simulink model "main_sim_generalized"  (R2024a)
settings: Solver=VariableStepAuto  StartTime=0.0  StopTime=Tsim  FixedStep=simStepSize  RelTol=1e-3
undefined symbols (not defined in the file): A_amp, B_para, f_d, f_hz, ForceDist, L_t, mmp_fir_coeff, mmp_iir_coeff, p_off, Ps_sys, Pz_sys, Qcvx_FIR, Qcvx_IIR, Qcvx_sim, SensorNoise, T_cs, T_fs, T_ss, Ts, Tu, w_k, w_k_IIR
libraries: cstblocks x6
settings Model: Creator=tomli  LastModifiedBy=tomli
settings RTWCC: GPUComputeCapability=3.5

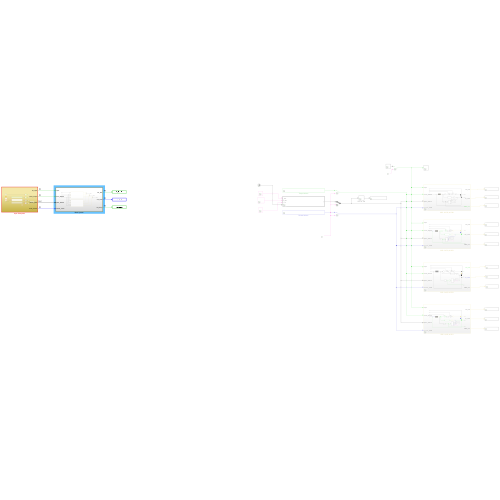
[thumbnail: Simulink's stored preview of the top-level diagram]
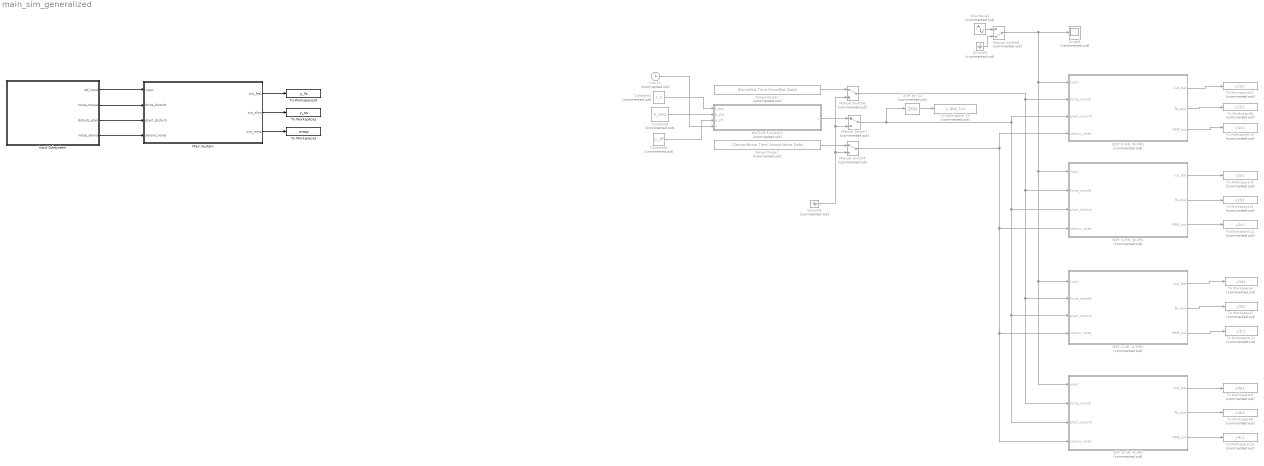
== system main_sim_generalized ==
  Clock1 : Clock  Commented=on
  Constant1 : Constant  Commented=on  Value=f_d
  Constant2 : Constant  Commented=on  Value=A_amp
  Constant3 : Constant  Commented=on  Value=p_off
  Ground3 : Ground  Commented=on
  Ground4 : Ground  Commented=on
  Input Subsystem : Subsystem
  MATLAB Function1 : MATLAB Function  Commented=on  TreatAsAtomicUnit=on
  Main System : Subsystem
  Manual Switch4 : ManualSwitch  Commented=on
  Manual Switch6 : ManualSwitch  Commented=on
  Manual Switch7 : ManualSwitch  Commented=on
  Manual Switch8 : ManualSwitch  Commented=on  CurrentSetting=0
  "SDP: Q-FIR, W-FIR1" : Subsystem  Commented=on
  "SDP: Q-FIR, W-IIR1" : Subsystem  Commented=on
  "SDP: Q-IIR, W-FIR1" : Subsystem  Commented=on
  "SDP: Q-IIR, W-IIR1" : Subsystem  Commented=on
  Scope1 : Scope  Commented=on
  Sensor Noise1 : FromWorkspace  Commented=on  VariableName=[SensorNoise.Time,SensorNoise.Data]  SampleTime=SensorNoise.Ts  Interpolate=off  ZeroCross=off  OutputAfterFinalValue=Setting to zero
  Sine Wave1 : Sin  Commented=on  SampleTime=Ts
  To Workspace 10 : ToWorkspace  Commented=on  VariableName=y1c1  SaveFormat=Structure With Time  SampleTime=Tu
      settings: MaxDataPoints=Inf
  To Workspace 11 : ToWorkspace  Commented=on  VariableName=y3c1  SaveFormat=Structure With Time  SampleTime=Tu
      settings: MaxDataPoints=Inf
  To Workspace 12 : ToWorkspace  Commented=on  VariableName=y2c1  SaveFormat=Structure With Time  SampleTime=Tu
      settings: MaxDataPoints=Inf
  To Workspace 13 : ToWorkspace  Commented=on  VariableName=y_dist_Tu1  SaveFormat=Structure With Time  SampleTime=Tu
      settings: MaxDataPoints=Inf
  To Workspace 14 : ToWorkspace  Commented=on  VariableName=y4c1  SaveFormat=Structure With Time  SampleTime=Tu
      settings: MaxDataPoints=Inf
  To Workspace 8 : ToWorkspace  Commented=on  VariableName=y2a1  SaveFormat=Structure With Time  SampleTime=Tu
      settings: MaxDataPoints=Inf
  To Workspace 9 : ToWorkspace  Commented=on  VariableName=y4a1  SaveFormat=Structure With Time  SampleTime=Tu
      settings: MaxDataPoints=Inf
  To Workspace1 : ToWorkspace  VariableName=y_ss  SaveFormat=Structure With Time  SampleTime=-1
  To Workspace10 : ToWorkspace  VariableName=y_fs  SaveFormat=Structure With Time  SampleTime=-1
  To Workspace11 : ToWorkspace  Commented=on  VariableName=y2b1  SaveFormat=Structure With Time  SampleTime=Ts
  To Workspace12 : ToWorkspace  Commented=on  VariableName=y1a1  SaveFormat=Structure With Time  SampleTime=-1
  To Workspace2 : ToWorkspace  VariableName=mmp  SaveFormat=Structure With Time  SampleTime=-1
  To Workspace4 : ToWorkspace  Commented=on  VariableName=y3a1  SaveFormat=Structure With Time  SampleTime=-1
  To Workspace6 : ToWorkspace  Commented=on  VariableName=y1b1  SaveFormat=Structure With Time  SampleTime=-1
  To Workspace7 : ToWorkspace  Commented=on  VariableName=y3b1  SaveFormat=Structure With Time  SampleTime=-1
  To Workspace8 : ToWorkspace  Commented=on  VariableName=y4b1  SaveFormat=Structure With Time  SampleTime=Ts
  Torque Noise1 : FromWorkspace  Commented=on  VariableName=[ForceDist.Time,ForceDist.Data]  SampleTime=ForceDist.Ts  Interpolate=off  ZeroCross=off  OutputAfterFinalValue=Setting to zero
  ZOH at Tu2 : ZeroOrderHold  Commented=on  SampleTime=Tu
  wires:
  Sensor Noise1/1 -> Manual Switch4/1
  "SDP: Q-IIR, W-FIR1"/2(fb_slow) -> To Workspace7/1
  Manual Switch7/1 -> ZOH at Tu2/1, "SDP: Q-IIR, W-IIR1"/3(plant_disturb), "SDP: Q-IIR, W-FIR1"/3(plant_disturb), "SDP: Q-FIR, W-IIR1"/3(plant_disturb), "SDP: Q-FIR, W-FIR1"/3(plant_disturb)
  Manual Switch4/1 -> "SDP: Q-FIR, W-FIR1"/4(sensor_noise), "SDP: Q-IIR, W-IIR1"/4(sensor_noise), "SDP: Q-IIR, W-FIR1"/4(sensor_noise), "SDP: Q-FIR, W-IIR1"/4(sensor_noise)
  "SDP: Q-IIR, W-IIR1"/2(fb_slow) -> To Workspace8/1
  "SDP: Q-FIR, W-FIR1"/2(fb_slow) -> To Workspace6/1
  "SDP: Q-FIR, W-FIR1"/3(MMP_out) -> To Workspace 10/1
  Torque Noise1/1 -> Manual Switch6/1
  Sine Wave1/1 -> Manual Switch8/1
  MATLAB Function1/1(y) -> Manual Switch7/1
  Manual Switch8/1 -> "SDP: Q-IIR, W-IIR1"/1(input), "SDP: Q-IIR, W-FIR1"/1(input), "SDP: Q-FIR, W-IIR1"/1(input), "SDP: Q-FIR, W-FIR1"/1(input), Scope1/1
  "SDP: Q-IIR, W-FIR1"/1(out_fast) -> To Workspace4/1
  "SDP: Q-IIR, W-IIR1"/3(MMP_out) -> To Workspace 14/1
  "SDP: Q-FIR, W-FIR1"/1(out_fast) -> To Workspace12/1
  "SDP: Q-IIR, W-IIR1"/1(out_fast) -> To Workspace 9/1
  Ground4/1 -> Manual Switch8/2
  ZOH at Tu2/1 -> To Workspace 13/1
  "SDP: Q-FIR, W-IIR1"/1(out_fast) -> To Workspace 8/1
  Constant1/1 -> MATLAB Function1/1(f_dist)
  Constant2/1 -> MATLAB Function1/2(A_dist)
  Ground3/1 -> Manual Switch6/2, Manual Switch7/2, Manual Switch4/2
  Clock1/1 -> MATLAB Function1/4(u)
  "SDP: Q-FIR, W-IIR1"/3(MMP_out) -> To Workspace 12/1
  Manual Switch6/1 -> "SDP: Q-IIR, W-IIR1"/2(force_disturb), "SDP: Q-IIR, W-FIR1"/2(force_disturb), "SDP: Q-FIR, W-IIR1"/2(force_disturb), "SDP: Q-FIR, W-FIR1"/2(force_disturb)
  Constant3/1 -> MATLAB Function1/3(p_off)
  "SDP: Q-IIR, W-FIR1"/3(MMP_out) -> To Workspace 11/1
  "SDP: Q-FIR, W-IIR1"/2(fb_slow) -> To Workspace11/1
  Input Subsystem/1(ref_input) -> Main System/1(input)
  Input Subsystem/2(noise_torque) -> Main System/2(force_disturb)
  Input Subsystem/3(disturb_plant) -> Main System/3(plant_disturb)
  Input Subsystem/4(noise_sensor) -> Main System/4(sensor_noise)
  Main System/3(out_mmp) -> To Workspace2/1
  Main System/2(out_slow) -> To Workspace1/1
  Main System/1(out_fast) -> To Workspace10/1

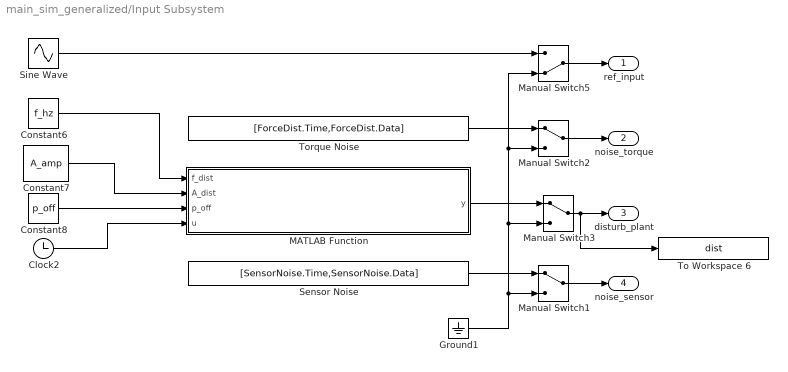
== system main_sim_generalized/Input Subsystem ==
  Clock2 : Clock
  Constant6 : Constant  Value=f_hz
  Constant7 : Constant  Value=A_amp
  Constant8 : Constant  Value=p_off
  Ground1 : Ground
  MATLAB Function : MATLAB Function  TreatAsAtomicUnit=on
  Manual Switch1 : ManualSwitch
  Manual Switch2 : ManualSwitch
  Manual Switch3 : ManualSwitch
  Manual Switch5 : ManualSwitch  CurrentSetting=0
  Sensor Noise : FromWorkspace  VariableName=[SensorNoise.Time,SensorNoise.Data]  SampleTime=SensorNoise.Ts  Interpolate=off  ZeroCross=off  OutputAfterFinalValue=Setting to zero
  Sine Wave : Sin  SampleTime=T_fs
  To Workspace 6 : ToWorkspace  VariableName=dist  SaveFormat=Structure With Time  SampleTime=T_fs
      settings: MaxDataPoints=Inf
  Torque Noise : FromWorkspace  VariableName=[ForceDist.Time,ForceDist.Data]  SampleTime=ForceDist.Ts  Interpolate=off  ZeroCross=off  OutputAfterFinalValue=Setting to zero
  ref_input : Outport
  noise_torque : Outport  Port=2
  disturb_plant : Outport  Port=3
  noise_sensor : Outport  Port=4
  wires:
  Manual Switch1/1 -> noise_sensor/1
  Constant7/1 -> MATLAB Function/2(A_dist)
  Constant8/1 -> MATLAB Function/3(p_off)
  Torque Noise/1 -> Manual Switch2/1
  Ground1/1 -> Manual Switch5/2, Manual Switch2/2, Manual Switch3/2, Manual Switch1/2
  Manual Switch3/1 -> To Workspace 6/1, disturb_plant/1
  Constant6/1 -> MATLAB Function/1(f_dist)
  Sine Wave/1 -> Manual Switch5/1
  MATLAB Function/1(y) -> Manual Switch3/1
  Clock2/1 -> MATLAB Function/4(u)
  Sensor Noise/1 -> Manual Switch1/1
  Manual Switch2/1 -> noise_torque/1
  Manual Switch5/1 -> ref_input/1

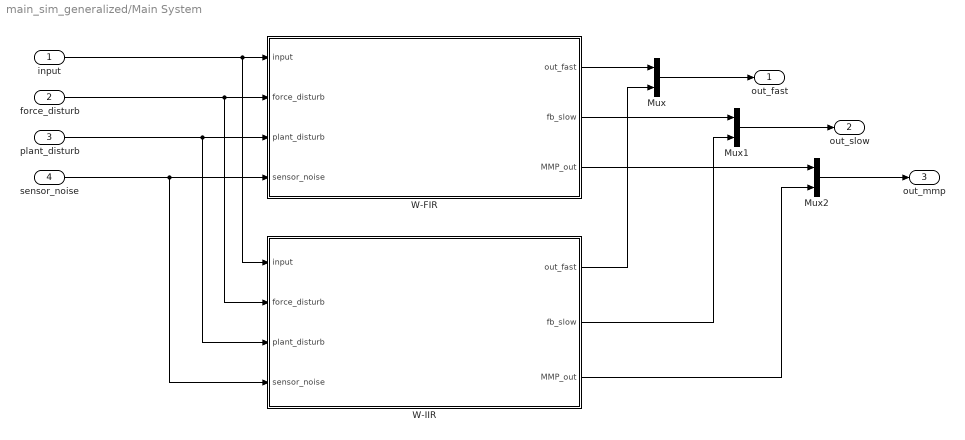
== system main_sim_generalized/Main System ==
  input : Inport
  force_disturb : Inport  Port=2
  plant_disturb : Inport  Port=3
  sensor_noise : Inport  Port=4
  Mux : Mux  Inputs=2
  Mux1 : Mux  Inputs=2
  Mux2 : Mux  Inputs=2
  W-FIR : Subsystem
  W-IIR : Subsystem
  out_fast : Outport
  out_slow : Outport  Port=2
  out_mmp : Outport  Port=3
  wires:
  W-FIR/2(fb_slow) -> Mux1/1
  plant_disturb/1 -> W-IIR/3(plant_disturb), W-FIR/3(plant_disturb)
  W-IIR/2(fb_slow) -> Mux1/2
  Mux1/1 -> out_slow/1
  W-IIR/1(out_fast) -> Mux/2
  sensor_noise/1 -> W-IIR/4(sensor_noise), W-FIR/4(sensor_noise)
  W-FIR/1(out_fast) -> Mux/1
  Mux/1 -> out_fast/1
  Mux2/1 -> out_mmp/1
  force_disturb/1 -> W-IIR/2(force_disturb), W-FIR/2(force_disturb)
  W-FIR/3(MMP_out) -> Mux2/1
  input/1 -> W-IIR/1(input), W-FIR/1(input)
  W-IIR/3(MMP_out) -> Mux2/2

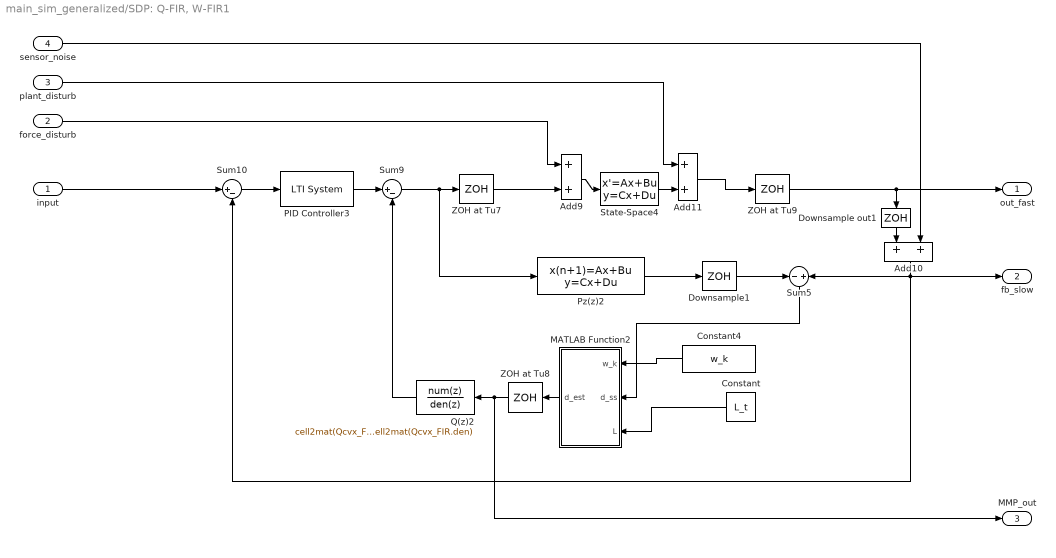
== system main_sim_generalized/SDP: Q-FIR, W-FIR1 ==
  input : Inport
  force_disturb : Inport  Port=2
  plant_disturb : Inport  Port=3
  sensor_noise : Inport  Port=4
  Add10 : Sum
  Add11 : Sum
  Add9 : Sum
  Constant : Constant  Value=L_t
  Constant4 : Constant  Value=w_k
  Downsample out1 : ZeroOrderHold  SampleTime=Ts
  Downsample1 : ZeroOrderHold  SampleTime=Ts
  MATLAB Function2 : MATLAB Function  TreatAsAtomicUnit=on  SystemSampleTime=T_cs
  PID Controller3 : cstblocks/LTI System  sys=Cz  IC=[]  PadeOrder=0
  Pz(z)2 : DiscreteStateSpace  A=Pz_sys.A  B=Pz_sys.B  C=Pz_sys.C  D=Pz_sys.D  SampleTime=Tu
  Q(z)2 : DiscreteTransferFcn  Numerator=cell2mat(Qcvx_FIR.num)  Denominator=cell2mat(Qcvx_FIR.den)  SampleTime=Tu
  State-Space4 : StateSpace  A=Ps_sys.A  B=Ps_sys.B  C=Ps_sys.C  D=Ps_sys.D  InitialCondition=0
  Sum10 : Sum  Inputs=|+-
  Sum5 : Sum  Inputs=-|+
  Sum9 : Sum  Inputs=|+-
  ZOH at Tu7 : ZeroOrderHold  SampleTime=Tu
  ZOH at Tu8 : ZeroOrderHold  SampleTime=Tu
  ZOH at Tu9 : ZeroOrderHold  SampleTime=Tu
  out_fast : Outport
  fb_slow : Outport  Port=2
  MMP_out : Outport  Port=3
  wires:
  ZOH at Tu9/1 -> Downsample out1/1, out_fast/1
  Sum9/1 -> Pz(z)2/1, ZOH at Tu7/1
  State-Space4/1 -> Add11/2
  Constant4/1 -> MATLAB Function2/1(w_k)
  Add10/1 -> Sum5/2, Sum10/2, fb_slow/1
  MATLAB Function2/1(d_est) -> ZOH at Tu8/1
  Add11/1 -> ZOH at Tu9/1
  force_disturb/1 -> Add9/1
  input/1 -> Sum10/1
  Pz(z)2/1 -> Downsample1/1
  ZOH at Tu8/1 -> MMP_out/1, Q(z)2/1
  Sum10/1 -> PID Controller3/1
  Add9/1 -> State-Space4/1
  Q(z)2/1 -> Sum9/2
  ZOH at Tu7/1 -> Add9/2
  Downsample1/1 -> Sum5/1
  Constant/1 -> MATLAB Function2/3(L)
  plant_disturb/1 -> Add11/1
  sensor_noise/1 -> Add10/2
  Downsample out1/1 -> Add10/1
  Sum5/1 -> MATLAB Function2/2(d_ss)
  PID Controller3/1 -> Sum9/1

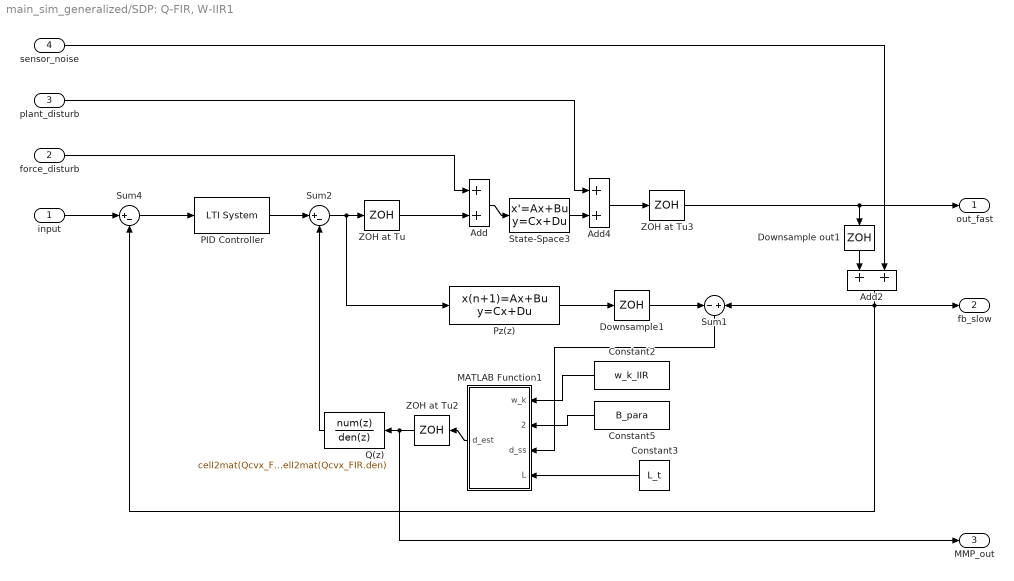
== system main_sim_generalized/SDP: Q-FIR, W-IIR1 ==
  input : Inport
  force_disturb : Inport  Port=2
  plant_disturb : Inport  Port=3
  sensor_noise : Inport  Port=4
  Add : Sum
  Add2 : Sum
  Add4 : Sum
  Constant2 : Constant  Value=w_k_IIR
  Constant3 : Constant  Value=L_t
  Constant5 : Constant  Value=B_para
  Downsample out1 : ZeroOrderHold  SampleTime=Ts
  Downsample1 : ZeroOrderHold  SampleTime=Ts
  MATLAB Function1 : MATLAB Function  TreatAsAtomicUnit=on  SystemSampleTime=T_cs
  PID Controller : cstblocks/LTI System  sys=Cz  IC=[]  PadeOrder=0
  Pz(z) : DiscreteStateSpace  A=Pz_sys.A  B=Pz_sys.B  C=Pz_sys.C  D=Pz_sys.D  SampleTime=Tu
  Q(z) : DiscreteTransferFcn  Numerator=cell2mat(Qcvx_FIR.num)  Denominator=cell2mat(Qcvx_FIR.den)  SampleTime=Tu
  State-Space3 : StateSpace  A=Ps_sys.A  B=Ps_sys.B  C=Ps_sys.C  D=Ps_sys.D  InitialCondition=0
  Sum1 : Sum  Inputs=-|+
  Sum2 : Sum  Inputs=|+-
  Sum4 : Sum  Inputs=|+-
  ZOH at Tu : ZeroOrderHold  SampleTime=Tu
  ZOH at Tu2 : ZeroOrderHold  SampleTime=Tu
  ZOH at Tu3 : ZeroOrderHold  SampleTime=Tu
  out_fast : Outport
  fb_slow : Outport  Port=2
  MMP_out : Outport  Port=3
  wires:
  Pz(z)/1 -> Downsample1/1
  ZOH at Tu/1 -> Add/2
  Add2/1 -> Sum1/2, Sum4/2, fb_slow/1
  Sum4/1 -> PID Controller/1
  State-Space3/1 -> Add4/2
  Downsample1/1 -> Sum1/1
  ZOH at Tu3/1 -> Downsample out1/1, out_fast/1
  Add4/1 -> ZOH at Tu3/1
  ZOH at Tu2/1 -> Q(z)/1, MMP_out/1
  Add/1 -> State-Space3/1
  Sum2/1 -> Pz(z)/1, ZOH at Tu/1
  Q(z)/1 -> Sum2/2
  force_disturb/1 -> Add/1
  plant_disturb/1 -> Add4/1
  sensor_noise/1 -> Add2/2
  input/1 -> Sum4/1
  Downsample out1/1 -> Add2/1
  Constant5/1 -> MATLAB Function1/2(B_para)
  Constant2/1 -> MATLAB Function1/1(w_k)
  MATLAB Function1/1(d_est) -> ZOH at Tu2/1
  Sum1/1 -> MATLAB Function1/3(d_ss)
  Constant3/1 -> MATLAB Function1/4(L)
  PID Controller/1 -> Sum2/1

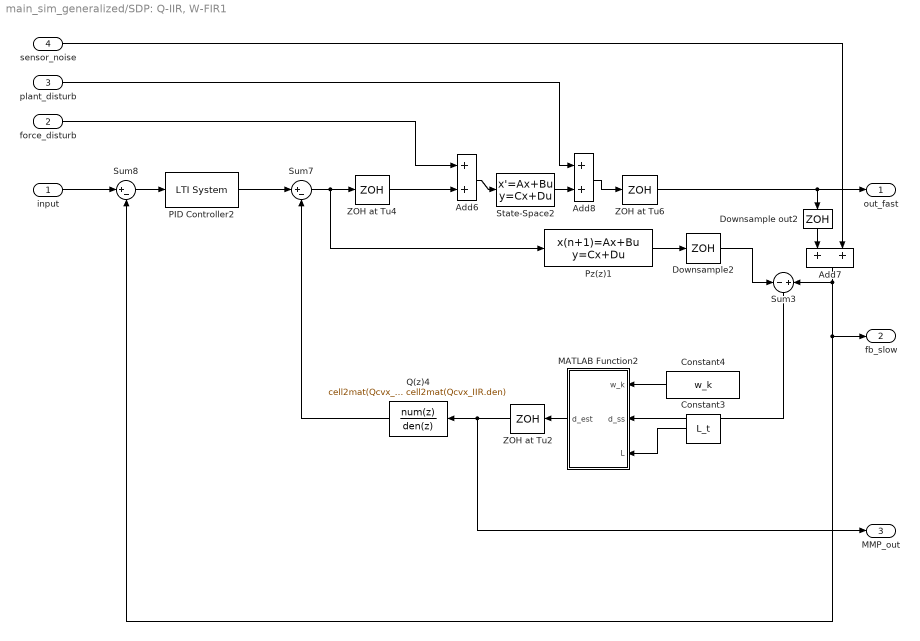
== system main_sim_generalized/SDP: Q-IIR, W-FIR1 ==
  input : Inport
  force_disturb : Inport  Port=2
  plant_disturb : Inport  Port=3
  sensor_noise : Inport  Port=4
  Add6 : Sum
  Add7 : Sum
  Add8 : Sum
  Constant3 : Constant  Value=L_t
  Constant4 : Constant  Value=w_k
  Downsample out2 : ZeroOrderHold  SampleTime=Ts
  Downsample2 : ZeroOrderHold  SampleTime=Ts
  MATLAB Function2 : MATLAB Function  TreatAsAtomicUnit=on  SystemSampleTime=T_cs
  PID Controller2 : cstblocks/LTI System  sys=Cz  IC=[]  PadeOrder=0
  Pz(z)1 : DiscreteStateSpace  A=Pz_sys.A  B=Pz_sys.B  C=Pz_sys.C  D=Pz_sys.D  SampleTime=Tu
  Q(z)4 : DiscreteTransferFcn  Numerator=cell2mat(Qcvx_IIR.num)  Denominator=cell2mat(Qcvx_IIR.den)
  State-Space2 : StateSpace  A=Ps_sys.A  B=Ps_sys.B  C=Ps_sys.C  D=Ps_sys.D  InitialCondition=0
  Sum3 : Sum  Inputs=-|+
  Sum7 : Sum  Inputs=|+-
  Sum8 : Sum  Inputs=|+-
  ZOH at Tu2 : ZeroOrderHold  SampleTime=Tu
  ZOH at Tu4 : ZeroOrderHold  SampleTime=Tu
  ZOH at Tu6 : ZeroOrderHold  SampleTime=Tu
  out_fast : Outport
  fb_slow : Outport  Port=2
  MMP_out : Outport  Port=3
  wires:
  Downsample2/1 -> Sum3/1
  Add8/1 -> ZOH at Tu6/1
  ZOH at Tu6/1 -> out_fast/1, Downsample out2/1
  ZOH at Tu4/1 -> Add6/2
  Add7/1 -> fb_slow/1, Sum8/2, Sum3/2
  input/1 -> Sum8/1
  sensor_noise/1 -> Add7/2
  Add6/1 -> State-Space2/1
  Sum8/1 -> PID Controller2/1
  State-Space2/1 -> Add8/2
  Sum7/1 -> Pz(z)1/1, ZOH at Tu4/1
  Pz(z)1/1 -> Downsample2/1
  plant_disturb/1 -> Add8/1
  force_disturb/1 -> Add6/1
  Downsample out2/1 -> Add7/1
  PID Controller2/1 -> Sum7/1
  Q(z)4/1 -> Sum7/2
  MATLAB Function2/1(d_est) -> ZOH at Tu2/1
  Sum3/1 -> MATLAB Function2/2(d_ss)
  ZOH at Tu2/1 -> MMP_out/1, Q(z)4/1
  Constant4/1 -> MATLAB Function2/1(w_k)
  Constant3/1 -> MATLAB Function2/3(L)

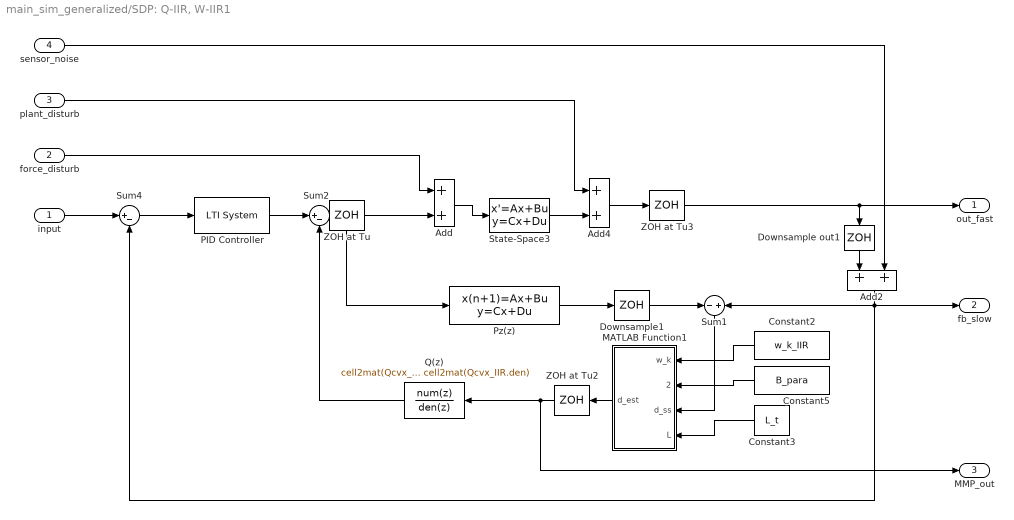
== system main_sim_generalized/SDP: Q-IIR, W-IIR1 ==
  input : Inport
  force_disturb : Inport  Port=2
  plant_disturb : Inport  Port=3
  sensor_noise : Inport  Port=4
  Add : Sum
  Add2 : Sum
  Add4 : Sum
  Constant2 : Constant  Value=w_k_IIR
  Constant3 : Constant  Value=L_t
  Constant5 : Constant  Value=B_para
  Downsample out1 : ZeroOrderHold  SampleTime=Ts
  Downsample1 : ZeroOrderHold  SampleTime=Ts
  MATLAB Function1 : MATLAB Function  TreatAsAtomicUnit=on  SystemSampleTime=T_cs
  PID Controller : cstblocks/LTI System  sys=Cz  IC=[]  PadeOrder=0
  Pz(z) : DiscreteStateSpace  A=Pz_sys.A  B=Pz_sys.B  C=Pz_sys.C  D=Pz_sys.D  SampleTime=Tu
  Q(z) : DiscreteTransferFcn  Numerator=cell2mat(Qcvx_IIR.num)  Denominator=cell2mat(Qcvx_IIR.den)  SampleTime=Tu
  State-Space3 : StateSpace  A=Ps_sys.A  B=Ps_sys.B  C=Ps_sys.C  D=Ps_sys.D  InitialCondition=0
  Sum1 : Sum  Inputs=-|+
  Sum2 : Sum  Inputs=|+-
  Sum4 : Sum  Inputs=|+-
  ZOH at Tu : ZeroOrderHold  SampleTime=Tu
  ZOH at Tu2 : ZeroOrderHold  SampleTime=Tu
  ZOH at Tu3 : ZeroOrderHold  SampleTime=Tu
  out_fast : Outport
  fb_slow : Outport  Port=2
  MMP_out : Outport  Port=3
  wires:
  ZOH at Tu/1 -> Add/2
  Add2/1 -> Sum1/2, Sum4/2, fb_slow/1
  Sum4/1 -> PID Controller/1
  State-Space3/1 -> Add4/2
  ZOH at Tu3/1 -> Downsample out1/1, out_fast/1
  Add4/1 -> ZOH at Tu3/1
  Add/1 -> State-Space3/1
  Sum2/1 -> Pz(z)/1, ZOH at Tu/1
  Q(z)/1 -> Sum2/2
  force_disturb/1 -> Add/1
  plant_disturb/1 -> Add4/1
  sensor_noise/1 -> Add2/2
  input/1 -> Sum4/1
  Downsample out1/1 -> Add2/1
  Constant5/1 -> MATLAB Function1/2(B_para)
  Constant2/1 -> MATLAB Function1/1(w_k)
  MATLAB Function1/1(d_est) -> ZOH at Tu2/1
  Sum1/1 -> MATLAB Function1/3(d_ss)
  Constant3/1 -> MATLAB Function1/4(L)
  Downsample1/1 -> Sum1/1
  Pz(z)/1 -> Downsample1/1
  ZOH at Tu2/1 -> Q(z)/1, MMP_out/1
  PID Controller/1 -> Sum2/1

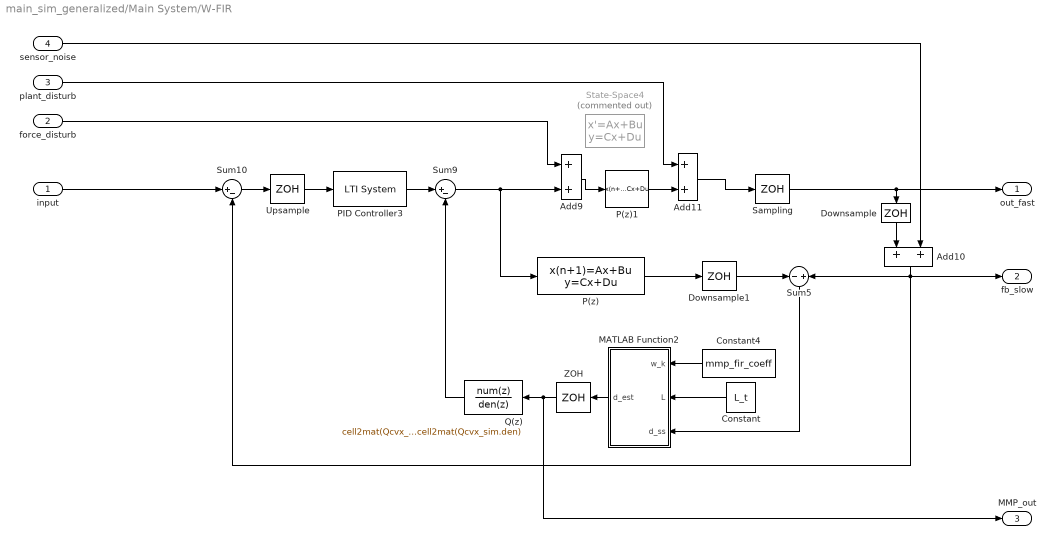
== system main_sim_generalized/Main System/W-FIR ==
  input : Inport
  force_disturb : Inport  Port=2
  plant_disturb : Inport  Port=3
  sensor_noise : Inport  Port=4
  Add10 : Sum
  Add11 : Sum
  Add9 : Sum
  Constant : Constant  Value=L_t
  Constant4 : Constant  Value=mmp_fir_coeff
  Downsample : ZeroOrderHold  SampleTime=T_ss
  Downsample1 : ZeroOrderHold  SampleTime=T_ss
  MATLAB Function2 : MATLAB Function  TreatAsAtomicUnit=on  SystemSampleTime=T_cs
  P(z) : DiscreteStateSpace  A=Pz_sys.A  B=Pz_sys.B  C=Pz_sys.C  D=Pz_sys.D  SampleTime=T_fs
  P(z)1 : DiscreteStateSpace  A=Pz_sys.A  B=Pz_sys.B  C=Pz_sys.C  D=Pz_sys.D  SampleTime=T_fs
  PID Controller3 : cstblocks/LTI System  sys=Cz  IC=[]  PadeOrder=0
  Q(z) : DiscreteTransferFcn  Numerator=cell2mat(Qcvx_sim.num)  Denominator=cell2mat(Qcvx_sim.den)  SampleTime=T_fs
  Sampling : ZeroOrderHold  SampleTime=T_fs
  State-Space4 : StateSpace  Commented=on  A=Ps_sys.A  B=Ps_sys.B  C=Ps_sys.C  D=Ps_sys.D  InitialCondition=0
  Sum10 : Sum  Inputs=|+-
  Sum5 : Sum  Inputs=-|+
  Sum9 : Sum  Inputs=|+-
  Upsample : ZeroOrderHold  SampleTime=T_fs
  ZOH : ZeroOrderHold  SampleTime=T_fs
  out_fast : Outport
  fb_slow : Outport  Port=2
  MMP_out : Outport  Port=3
  wires:
  Sampling/1 -> Downsample/1, out_fast/1
  P(z)1/1 -> Add11/2
  Constant4/1 -> MATLAB Function2/1(w_k)
  Add10/1 -> Sum5/2, Sum10/2, fb_slow/1
  MATLAB Function2/1(d_est) -> ZOH/1
  Add11/1 -> Sampling/1
  force_disturb/1 -> Add9/1
  input/1 -> Sum10/1
  P(z)/1 -> Downsample1/1
  ZOH/1 -> MMP_out/1, Q(z)/1
  Sum10/1 -> Upsample/1
  Add9/1 -> P(z)1/1
  Q(z)/1 -> Sum9/2
  Sum9/1 -> Add9/2, P(z)/1
  Downsample1/1 -> Sum5/1
  Constant/1 -> MATLAB Function2/2(L)
  plant_disturb/1 -> Add11/1
  sensor_noise/1 -> Add10/2
  Downsample/1 -> Add10/1
  Sum5/1 -> MATLAB Function2/3(d_ss)
  PID Controller3/1 -> Sum9/1
  Upsample/1 -> PID Controller3/1

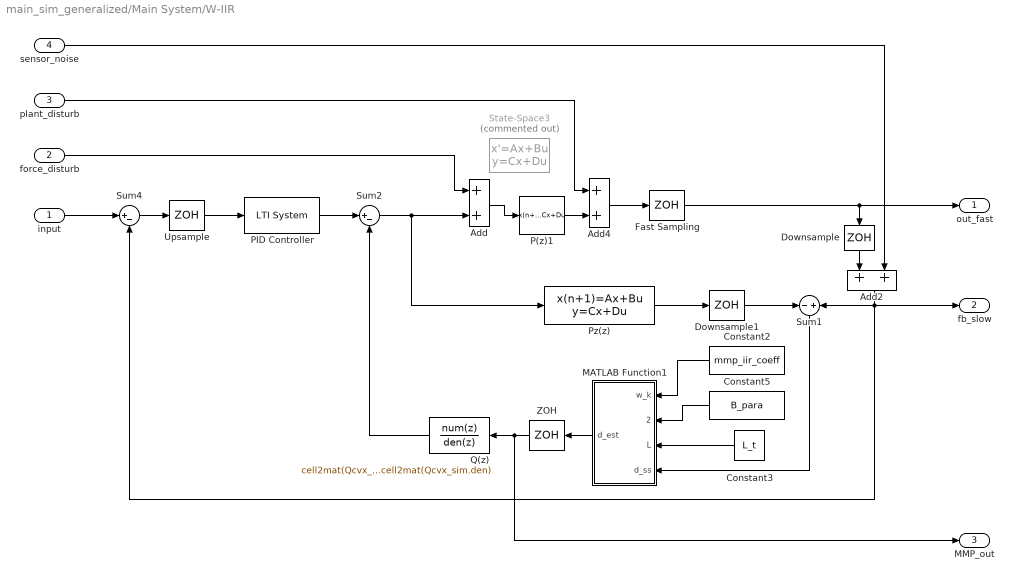
== system main_sim_generalized/Main System/W-IIR ==
  input : Inport
  force_disturb : Inport  Port=2
  plant_disturb : Inport  Port=3
  sensor_noise : Inport  Port=4
  Add : Sum
  Add2 : Sum
  Add4 : Sum
  Constant2 : Constant  Value=mmp_iir_coeff
  Constant3 : Constant  Value=L_t
  Constant5 : Constant  Value=B_para
  Downsample : ZeroOrderHold  SampleTime=T_ss
  Downsample1 : ZeroOrderHold  SampleTime=T_ss
  Fast Sampling : ZeroOrderHold  SampleTime=T_fs
  MATLAB Function1 : MATLAB Function  TreatAsAtomicUnit=on  SystemSampleTime=T_cs
  P(z)1 : DiscreteStateSpace  A=Pz_sys.A  B=Pz_sys.B  C=Pz_sys.C  D=Pz_sys.D  SampleTime=T_fs
  PID Controller : cstblocks/LTI System  sys=Cz  IC=[]  PadeOrder=0
  Pz(z) : DiscreteStateSpace  A=Pz_sys.A  B=Pz_sys.B  C=Pz_sys.C  D=Pz_sys.D  SampleTime=T_fs
  Q(z) : DiscreteTransferFcn  Numerator=cell2mat(Qcvx_sim.num)  Denominator=cell2mat(Qcvx_sim.den)  SampleTime=T_fs
  State-Space3 : StateSpace  Commented=on  A=Ps_sys.A  B=Ps_sys.B  C=Ps_sys.C  D=Ps_sys.D  InitialCondition=0
  Sum1 : Sum  Inputs=-|+
  Sum2 : Sum  Inputs=|+-
  Sum4 : Sum  Inputs=|+-
  Upsample : ZeroOrderHold  SampleTime=T_fs
  ZOH : ZeroOrderHold  SampleTime=T_fs
  out_fast : Outport
  fb_slow : Outport  Port=2
  MMP_out : Outport  Port=3
  wires:
  Pz(z)/1 -> Downsample1/1
  Sum2/1 -> Pz(z)/1, Add/2
  Add2/1 -> Sum1/2, Sum4/2, fb_slow/1
  Sum4/1 -> Upsample/1
  P(z)1/1 -> Add4/2
  Downsample1/1 -> Sum1/1
  Fast Sampling/1 -> Downsample/1, out_fast/1
  Add4/1 -> Fast Sampling/1
  ZOH/1 -> Q(z)/1, MMP_out/1
  Add/1 -> P(z)1/1
  Q(z)/1 -> Sum2/2
  force_disturb/1 -> Add/1
  plant_disturb/1 -> Add4/1
  sensor_noise/1 -> Add2/2
  input/1 -> Sum4/1
  Downsample/1 -> Add2/1
  Constant5/1 -> MATLAB Function1/2(B_para)
  Constant2/1 -> MATLAB Function1/1(w_k)
  MATLAB Function1/1(d_est) -> ZOH/1
  Sum1/1 -> MATLAB Function1/4(d_ss)
  Constant3/1 -> MATLAB Function1/3(L)
  PID Controller/1 -> Sum2/1
  Upsample/1 -> PID Controller/1

== matlab function main_sim_generalized/Input Subsystem/MATLAB Function ==
  data: f_dist input; A_dist input; p_off input; u input; y output
function y = fcn(f_dist,A_dist,p_off,u)
y = zeros(1,length(u));
for i = 1:length(f_dist)
y = y + A_dist(i)*sin(2*pi*f_dist(i)*u+p_off(i));
end

== matlab function main_sim_generalized/Main System/W-FIR/MATLAB Function2 ==
  settings: updateMethod=DISCRETE
  data: w_k input; L input; d_ss input; d_est output
% FIR siganl reconstruction
function d_est = fcn(w_k,L,d_ss)
persistent n_w phi n_fs n_ss n_cs N_L; % keeps data of variables

% assigning initial values
if isempty(n_w)
    n_w = size(w_k,1); % n_w = 2m disturbances (index starts at 0,1,...,2m-1)
    phi = zeros(1,n_w);
    n_fs = 0;
    n_ss = 0;
    n_cs = 0;
    [N_L, ~] = rat(L);
end

% starts first loop with n_fs = 1 and n_ss = 1
% in MATLAB, d_ss[n_ss] = d_fs[(n_ss-1)*L+1] % for n_ss = 1, ...
% counter for loops performed
n_cs = n_cs + 1; % # of combined samples, where D_L*T_cs = T_fs
n_fs = n_fs+1; % (# of fast samples)

k = mod((n_cs-1), N_L); % kth intersample point
if k == 0 % update number of slow samples
    n_ss = n_ss + 1; % number of slow samples
end

%% FIR-MMP cases
%% case 1: n_sl < 2*m (not enough data points for FIR)
% case 1 will update phi until there is 2*m slow measured data points
% phi[n] = d_sl[n], phi(1,2m) used to temporarily store the last 2*m ...
% ... measured data points
% 1a: n_sl < 2*m and k=0 means slow and fast measurements match ...
% ... d_sl [n_sl] = d[(n_sl-1)L+1].
% need to update the new set of data points needed to start reconstruction
if (n_ss<n_w) && (k==0)
    for i = 1:(n_w-1)
        phi(n_w-i+1) = phi(n_w-i); % shifts signal data phi(1) -> phi(2)
    end
    phi(1) = d_ss; % current measured data point
    d_est = d_ss; % set d_est = d_ss since the slow and fast align
% when k ~= 0, this is the intersample point, but there is not enough ...
% ... data points, keep this off
elseif (n_ss<n_w) && k~=0 % intersample point estimation
    d_est = 0;
%% case 2: n_ss >= 2m (enough data points for FIR)
% enough data points exist for FIR signal reconstruction
elseif (n_ss>=n_w) && k==0
    for i = 1:(n_w-1)
        phi(n_w-i+1) = phi(n_w-i);
    end
    phi(1) = d_ss;
    d_est = d_ss;
else % final case: n_ss >= n_w && k~=0
    d_est = phi*w_k(:,k); % signal reconstruction step
end

== matlab function main_sim_generalized/Main System/W-IIR/MATLAB Function1 ==
  settings: updateMethod=DISCRETE
  data: w_k input; B_para input; L input; d_ss input; d_est output
% IIR signal reconstruction
function d_est = fcn(w_k, B_para, L, d_ss) % keeps data of variables
persistent phi n_cs n_ss N_L n_w d_buff max_buffer_size buffer_indices;

% assigning initial values
if isempty(n_w)
    n_w = size(w_k,1); % n_w = 2m disturbances (index starts at 0,1,...,2m-1)
    phi = zeros(1,n_w);
    n_ss = 0;
    n_cs = 0;
    % d_IIR = zeros(1,0); % stored fast sampling signal
    [N_L, ~] = rat(L);
    buffer_indices = 2:N_L:((n_w-1) * N_L + 2);
    max_buffer_size = (n_w * N_L + 1);
    d_buff = zeros(1, max_buffer_size, 'like', d_ss);
end

% starts first loop with n_fs = 1 and n_ss = 1
% in MATLAB, d_ss[n_ss] = d_fs[(n_ss-1)*L+1] % for n_ss = 1, ...
% counter for loops performed
n_cs = n_cs + 1;
k = mod((n_cs-1), N_L);
if k == 0 % update number of slow samples
    n_ss = n_ss + 1; % number of slow samples
end

%% MMP IIR reconstruction cases
%% case 1: n_sl < 2*m (not enough data points for FIR)
% case 1 will update phi until there is 2*m slow measured data points
% phi[n] = d_sl[n], phi(1,2m) used to temporarily store the last 2*m ...
% ... measured data points
% 1a: n_sl < 2*m and k=0 means slow and fast measurements match ...
% ... d_sl [n_sl] = d[(n_sl-1)L+1].
% need to update the new set of data points needed to start reconstruction
if (n_ss < n_w) && (k==0)
    for i = 1:(n_w-1)
        phi(n_w-i+1) = phi(n_w-i); % shifts signal data phi(1) -> phi(2)
    end
    phi(1) = d_ss; % current measured data point
    d_est = d_ss; % set d_est = d_ss since the slow and fast align
    d_buff = [d_est, d_buff(1:end-1)];
% when k ~= 0, this is the intersample point, but there is not enough ...
% ... data points, keep this off
% elseif (n_ss < n_w) && (k~=0) % intersample point estimation
elseif (n_ss < n_w) && (k~=0) % intersample point estimation
    d_est = 0;
    d_buff = [d_est, d_buff(1:end-1)];
%% case 2: n_sl >= 2m (enough data points for FIR)
% enough data points exist to start FIR signal reconstruction
elseif  (n_ss >= n_w) && (n_ss < (n_w+1)) && (k==0) 
    for i = 1:(n_w-1)
        phi(n_w-i+1) = phi(n_w-i);
    end
    phi(1) = d_ss;
    d_est = d_ss;
    d_buff = [d_est, d_buff(1:end-1)];
elseif (n_ss >= n_w) && (n_ss < (n_w+1)) && (k~=0) % intersmaple point
    d_est = 0;
    d_buff = [d_est, d_buff(1:end-1)];
%% case 3: n_sl >= 2m+1 (enough data points for IIR)
elseif (n_ss >= (n_w+1)) && k==0
    for i = 1:(n_w-1)
        phi(n_w-i+1) = phi(n_w-i);
    end
    phi(1) = d_ss;
    d_est = d_ss;
    d_buff = [d_est, d_buff(1:end-1)];
else % n_ss>=(n_w+1) && k~=0
    d_temp = flip(d_buff);
    d_est = phi * w_k(:,k) - ...
            d_temp(buffer_indices) * flip(B_para(2:end));
    d_buff = [d_est, d_buff(1:end-1)];
end

== matlab function main_sim_generalized/MATLAB Function1 ==
  data: f_dist input; A_dist input; p_off input; u input; y output
function y = fcn(f_dist,A_dist,p_off,u)
y = zeros(1,length(u));
for i = 1:length(f_dist)
y = y + A_dist(i)*sin(2*pi*f_dist(i)*u+p_off(i));
end

== matlab function main_sim_generalized/SDP: Q-FIR, W-FIR1/MATLAB Function2 ==
  settings: updateMethod=DISCRETE
  data: w_k input; d_ss input; L input; d_est output
% FIR siganl reconstruction
function d_est = fcn(w_k,d_ss,L)
persistent n_w phi n_fs n_ss n_cs N_L; % keeps data of variables
% assigning initial values
if isempty(n_w)
    n_w = size(w_k,1); % n_w = 2m disturbances (index starts at 0,1,...,2m-1)
    phi = zeros(1,n_w);
    n_fs = 0;
    n_ss = 0;
    n_cs = 0;
    [N_L, ~] = rat(L);
end

% starts first loop with n_fs = 1 and n_ss = 1
% in MATLAB, d_ss[n_ss] = d_fs[(n_ss-1)*L+1] % for n_ss = 1, ...
% counter for loops performed
n_cs = n_cs + 1; % # of combined samples, where D_L*T_cs = T_fs
n_fs = n_fs+1; % (# of fast samples)

k = mod((n_cs-1), N_L); % kth intersample point
if k == 0 % update number of slow samples
    n_ss = n_ss + 1; % number of slow samples
end

%% case 1: n_sl < 2*m (not enough data points for FIR)
% case 1 will update phi until there is 2*m slow measured data points
% phi[n] = d_sl[n], phi(1,2m) used to temporarily store the last 2*m ...
% ... measured data points
% 1a: n_sl < 2*m and k=0 means slow and fast measurements match ...
% ... d_sl [n_sl] = d[(n_sl-1)L+1].
% need to update the new set of data points needed to start reconstruction
if (n_ss<n_w) && (k==0)
    for i = 1:(n_w-1)
    phi(n_w-i+1) = phi(n_w-i); % shifts signal data phi(1) -> phi(2)
    end
    phi(1) = d_ss; % current measured data point
    d_est = d_ss; % set d_est = d_ss since the slow and fast align
% when k ~= 0, this is the intersample point, but there is not enough ...
% ... data points, keep this off
elseif (n_ss<n_w) && k~=0 % intersample point estimation
    d_est = 0;
%% case 2: n_ss >= 2m (enough data points for FIR)
% enough data points exist for FIR signal reconstruction
elseif (n_ss>=n_w) && k==0
    for i = 1:(n_w-1)
    phi(n_w-i+1) = phi(n_w-i);
    end
    phi(1) = d_ss;
    d_est = d_ss;
else % final case: n_ss >= n_w && k~=0
    d_est = phi*w_k(:,k); % signal reconstruction step
end

== matlab function main_sim_generalized/SDP: Q-FIR, W-IIR1/MATLAB Function1 ==
  settings: updateMethod=DISCRETE
  data: w_k input; B_para input; d_ss input; L input; d_est output
% IIR signal reconstruction based on 2018 paper. Rejecting fast narrow-band
% disturbances with slow sensor feedback for quality beam steering in
% selective laser sintering (Xiao, H.; Jiang, T; Chen, X.)
function d_est = fcn(w_k, B_para, d_ss,L) % keeps data of variables
persistent phi n_cs n_ss d_IIR N_L n_w d_buff max_buffer_size buffer_indices;

% assigning initial values
if isempty(n_w)
    n_w = size(w_k,1); % n_w = 2m disturbances (index starts at 0,1,...,2m-1)
    phi = zeros(1,n_w);
    n_ss = 0;
    n_cs = 0;
    % d_IIR = zeros(1,0); % stored fast sampling signal
    [N_L, ~] = rat(L);
    buffer_indices = 2:N_L:((n_w-1) * N_L + 2);
    max_buffer_size = (n_w * N_L + 1);
    d_buff = zeros(1, max_buffer_size, 'like', d_ss);
end

% starts first loop with n_fs = 1 and n_ss = 1
% in MATLAB, d_ss[n_ss] = d_fs[(n_ss-1)*L+1] % for n_ss = 1, ...
% counter for loops performed
n_cs = n_cs + 1;
k = mod((n_cs-1), N_L);
if k == 0 % update number of slow samples
    n_ss = n_ss + 1; % number of slow samples
end

%% case 1: n_sl < 2*m (not enough data points for FIR)
% case 1 will update phi until there is 2*m slow measured data points
% phi[n] = d_sl[n], phi(1,2m) used to temporarily store the last 2*m ...
% ... measured data points
% 1a: n_sl < 2*m and k=0 means slow and fast measurements match ...
% ... d_sl [n_sl] = d[(n_sl-1)L+1].
% need to update the new set of data points needed to start reconstruction
if (n_ss < n_w) && (k==0)
    for i = 1:(n_w-1)
        phi(n_w-i+1) = phi(n_w-i); % shifts signal data phi(1) -> phi(2)
    end
    phi(1) = d_ss; % current measured data point
    d_est = d_ss; % set d_est = d_ss since the slow and fast align
    d_buff = [d_est, d_buff(1:end-1)];
    % d_IIR(end+1) = d_est;
% when k ~= 0, this is the intersample point, but there is not enough ...
% ... data points, keep this off
% elseif (n_ss < n_w) && (k~=0) % intersample point estimation
elseif (n_ss < n_w) && (k~=0) % intersample point estimation
    d_est = 0;
    d_buff = [d_est, d_buff(1:end-1)];
    % d_IIR(end+1) = d_est;
%% case 2: n_sl >= 2m (enough data points for FIR)
% enough data points exist to start FIR signal reconstruction
elseif  (n_ss >= n_w) && (n_ss < (n_w+1)) && (k==0) 
    for i = 1:(n_w-1)
        phi(n_w-i+1) = phi(n_w-i);
    end
    phi(1) = d_ss;
    d_est = d_ss;
    d_buff = [d_est, d_buff(1:end-1)];
    % d_IIR(end+1) = d_ss;
elseif (n_ss >= n_w) && (n_ss < (n_w+1)) && (k~=0) % intersmaple point
    % d_est = phi*w_k(:,k);
    d_est = 0;
    % d_IIR(end+1) = d_est;
    d_buff = [d_est, d_buff(1:end-1)];
%% case 3: n_sl >= 2m+1 (enough data points for IIR)
elseif (n_ss >= (n_w+1)) && k==0
    for i = 1:(n_w-1)
        phi(n_w-i+1) = phi(n_w-i);
    end
    phi(1) = d_ss;
    d_est = d_ss;
    % d_IIR(end+1) = d_est;
    d_buff = [d_est, d_buff(1:end-1)];
else % n_ss>=(n_w+1) && k~=0
    % d_est = phi*w_k(:,k)-...
    % flip(d_IIR(((n_ss-n_w-1)*N_L + k + 1):N_L:((n_ss-2)*N_L+k+1)))*B_para(2:end);
    % d_IIR(end+1) = d_est;
    d_temp = flip(d_buff);
    d_est = phi * w_k(:,k) - ...
            d_temp(buffer_indices) * flip(B_para(2:end));
    d_buff = [d_est, d_buff(1:end-1)];
end

== matlab function main_sim_generalized/SDP: Q-IIR, W-FIR1/MATLAB Function2 ==
  settings: updateMethod=DISCRETE
  data: w_k input; d_ss input; L input; d_est output
% FIR siganl reconstruction
function d_est = fcn(w_k,d_ss,L)
persistent n_w phi n_fs n_ss n_cs N_L; % keeps data of variables
% assigning initial values
if isempty(n_w)
    n_w = size(w_k,1); % n_w = 2m disturbances (index starts at 0,1,...,2m-1)
    phi = zeros(1,n_w);
    n_fs = 0;
    n_ss = 0;
    n_cs = 0;
    [N_L, ~] = rat(L);
end

% starts first loop with n_fs = 1 and n_ss = 1
% in MATLAB, d_ss[n_ss] = d_fs[(n_ss-1)*L+1] % for n_ss = 1, ...
% counter for loops performed
n_cs = n_cs + 1; % # of combined samples, where D_L*T_cs = T_fs
n_fs = n_fs+1; % (# of fast samples)

k = mod((n_cs-1), N_L); % kth intersample point
if k == 0 % update number of slow samples
    n_ss = n_ss + 1; % number of slow samples
end

%% case 1: n_sl < 2*m (not enough data points for FIR)
% case 1 will update phi until there is 2*m slow measured data points
% phi[n] = d_sl[n], phi(1,2m) used to temporarily store the last 2*m ...
% ... measured data points
% 1a: n_sl < 2*m and k=0 means slow and fast measurements match ...
% ... d_sl [n_sl] = d[(n_sl-1)L+1].
% need to update the new set of data points needed to start reconstruction
if (n_ss<n_w) && (k==0)
    for i = 1:(n_w-1)
    phi(n_w-i+1) = phi(n_w-i); % shifts signal data phi(1) -> phi(2)
    end
    phi(1) = d_ss; % current measured data point
    d_est = d_ss; % set d_est = d_ss since the slow and fast align
% when k ~= 0, this is the intersample point, but there is not enough ...
% ... data points, keep this off
elseif (n_ss<n_w) && k~=0 % intersample point estimation
    d_est = 0;
%% case 2: n_ss >= 2m (enough data points for FIR)
% enough data points exist for FIR signal reconstruction
elseif (n_ss>=n_w) && k==0
    for i = 1:(n_w-1)
    phi(n_w-i+1) = phi(n_w-i);
    end
    phi(1) = d_ss;
    d_est = d_ss;
else % final case: n_ss >= n_w && k~=0
    d_est = phi*w_k(:,k); % signal reconstruction step
end

== matlab function main_sim_generalized/SDP: Q-IIR, W-IIR1/MATLAB Function1 ==
  settings: updateMethod=DISCRETE
  data: w_k input; B_para input; d_ss input; L input; d_est output
% IIR signal reconstruction based on 2018 paper. Rejecting fast narrow-band
% disturbances with slow sensor feedback for quality beam steering in
% selective laser sintering (Xiao, H.; Jiang, T; Chen, X.)
function d_est = fcn(w_k, B_para, d_ss,L) % keeps data of variables
persistent phi n_cs n_ss d_IIR N_L n_w d_buff max_buffer_size buffer_indices;

% assigning initial values
if isempty(n_w)
    n_w = size(w_k,1); % n_w = 2m disturbances (index starts at 0,1,...,2m-1)
    phi = zeros(1,n_w);
    n_ss = 0;
    n_cs = 0;
    % d_IIR = zeros(1,0); % stored fast sampling signal
    [N_L, ~] = rat(L);
    buffer_indices = 2:N_L:((n_w-1) * N_L + 2);
    max_buffer_size = (n_w * N_L + 1);
    d_buff = zeros(1, max_buffer_size, 'like', d_ss);
end

% starts first loop with n_fs = 1 and n_ss = 1
% in MATLAB, d_ss[n_ss] = d_fs[(n_ss-1)*L+1] % for n_ss = 1, ...
% counter for loops performed
n_cs = n_cs + 1;
k = mod((n_cs-1), N_L);
if k == 0 % update number of slow samples
    n_ss = n_ss + 1; % number of slow samples
end

%% case 1: n_sl < 2*m (not enough data points for FIR)
% case 1 will update phi until there is 2*m slow measured data points
% phi[n] = d_sl[n], phi(1,2m) used to temporarily store the last 2*m ...
% ... measured data points
% 1a: n_sl < 2*m and k=0 means slow and fast measurements match ...
% ... d_sl [n_sl] = d[(n_sl-1)L+1].
% need to update the new set of data points needed to start reconstruction
if (n_ss < n_w) && (k==0)
    for i = 1:(n_w-1)
        phi(n_w-i+1) = phi(n_w-i); % shifts signal data phi(1) -> phi(2)
    end
    phi(1) = d_ss; % current measured data point
    d_est = d_ss; % set d_est = d_ss since the slow and fast align
    d_buff = [d_est, d_buff(1:end-1)];
    % d_IIR(end+1) = d_est;
% when k ~= 0, this is the intersample point, but there is not enough ...
% ... data points, keep this off
% elseif (n_ss < n_w) && (k~=0) % intersample point estimation
elseif (n_ss < n_w) && (k~=0) % intersample point estimation
    d_est = 0;
    d_buff = [d_est, d_buff(1:end-1)];
    % d_IIR(end+1) = d_est;
%% case 2: n_sl >= 2m (enough data points for FIR)
% enough data points exist to start FIR signal reconstruction
elseif  (n_ss >= n_w) && (n_ss < (n_w+1)) && (k==0) 
    for i = 1:(n_w-1)
        phi(n_w-i+1) = phi(n_w-i);
    end
    phi(1) = d_ss;
    d_est = d_ss;
    d_buff = [d_est, d_buff(1:end-1)];
    % d_IIR(end+1) = d_ss;
elseif (n_ss >= n_w) && (n_ss < (n_w+1)) && (k~=0) % intersmaple point
    % d_est = phi*w_k(:,k);
    d_est = 0;
    % d_IIR(end+1) = d_est;
    d_buff = [d_est, d_buff(1:end-1)];
%% case 3: n_sl >= 2m+1 (enough data points for IIR)
elseif (n_ss >= (n_w+1)) && k==0
    for i = 1:(n_w-1)
        phi(n_w-i+1) = phi(n_w-i);
    end
    phi(1) = d_ss;
    d_est = d_ss;
    % d_IIR(end+1) = d_est;
    d_buff = [d_est, d_buff(1:end-1)];
else % n_ss>=(n_w+1) && k~=0
    % d_est = phi*w_k(:,k)-...
    % flip(d_IIR(((n_ss-n_w-1)*N_L + k + 1):N_L:((n_ss-2)*N_L+k+1)))*B_para(2:end);
    % d_IIR(end+1) = d_est;
    d_temp = flip(d_buff);
    d_est = phi * w_k(:,k) - ...
            d_temp(buffer_indices) * flip(B_para(2:end));
    d_buff = [d_est, d_buff(1:end-1)];
end
